simulink model "unpack"  (R2018b)
settings: Solver=VariableStepAuto  StartTime=0.0  StopTime=10.0  RelTol=1e-3
(part 2 of 2)

== matlab function unpack/message_unpack ==
  data: CAFDva_y_F_RadarData151 input size=22; CAFDva_y_F_RadarData152 input size=50; CAFDva_y_F_RadarData153 input size=50; CAFDva_y_F_RadarData154 input size=50; CAFDva_y_F_RadarData155 input size=50; CAFDva_y_F_RadarData156 input size=50; CAFDva_y_F_RadarData157 input size=50; CAFDva_y_F_RadarData158 input size=50; CAFDva_y_F_RadarData159 input size=50; CAFDva_y_F_RadarData15A input size=50; CAFDva_y_F_RadarData15B input size=50; CAFDva_y_F_RadarData15C input size=50; CAFDva_y_F_RadarData15D input size=50; CAFDva_y_F_RadarData15E input size=50; CAFDva_y_F_RadarData15F input size=50; CAFDva_y_F_RadarData160 input size=50; CAFDva_y_F_RadarData161 input size=50; CAFDva_y_F_RadarData162 input size=50; CAFDva_y_F_RadarData163 input size=50; CAFDva_y_F_RadarData164 input size=50; CAFDva_y_F_RadarData165 input size=50; CAFDva_y_F_RadarData166 input size=50; CAFDva_y_F_RadarData167 input size=50; CAFDva_y_F_RadarData168 input size=50; CAFDva_y_F_RadarData169 input size=50; CAFDva_y_F_CameraData600 input; CAFDva_y_F_CameraData424 input; CAFDva_y_F_CameraData425 input; CAFDva_y_F_CameraData450 input; CAFDva_y_F_CameraData459 input; CAFDva_y_F_CameraData45A input; CAFDva_y_F_CameraData45B input; CAFDva_y_F_CameraData45C input; CAFDva_y_F_CameraData45D input; CAFDva_y_F_CameraData45E input; CAFDva_y_F_CameraData45F input; CAFDva_y_F_CameraData420 input; CAFDva_y_F_CameraData421 input; CAFDva_y_F_CameraData422 input; CAFDva_y_F_CameraData451 input; CAFDva_y_F_CameraData423 input; CAFDva_y_F_CameraData452 input; CAFDva_y_F_CameraData453 input; CAFDva_y_F_CameraData454 input; CAFDva_y_F_CameraData455 input; CAFDva_y_F_CameraData456 input; CAFDva_y_F_CameraData457 input; CAFDva_y_F_CameraData458 input; CAFDva_y_F_CameraData449 input; Rar_obj_timestamp output; Radar_Status output; Radar_num output; CorrCoeff_x_vx output; CorrCoeff_y_vy output; CorrCoeff_y_vx output; CorrCoeff_x_vy output; IsNew output; YawSTD output; YawAngle output; WidthSTD output; Width output; RadarCrossSection output single; MovementStatus output; LongDistanceSTD output; LengthSTD output; Length output; LateralDistanceSTD output; LatDistance output; ExistenceProb output; CorrCoeff_x_y output; ClassType output; ClassProbValue output; CorrCoeff_vx_vy output; AbsoluteLongVelo output; AbsoluteLongAcc output; AbsoluteLatVelo output; AbsoluteLatAcc output; AbsLongVeloSTD output; AbsLongAccSTD output; AbsLatVeloSTD output; AbsLatAccSTD output; LongDistance output; ReferencePoint output; MeasurementStatus output; ObjectAge output; ObjectID output; IFC_obj_timestamp output; IFC_State output; IFC_ObjHdr_ObjCount output; IFC_VD_CIPV_ID output; FS_Out_Of_Calib output uint8; FS_Rain output; FS_Fog output; FS_Splashes_0 output; FS_Sun_Ray_0 output; FS_Low_Sun_0 output; FS_Blur_Image_0 output; FS_Partial_Blockage_0 output; FS_Full_Blockage_0 output; FS_Frozen_Windshield_0 output; FS_Out_Of_Focus_0 output; IFC_obj_TTIPC_StdDev output single; IFC_obj_abs_Ax output single; IFC_obj_abs_Ay output single; IFC_obj_Rel_Vx output; IFC_obj_Rel_Vy output; IFC_obj_Dx output; IFC_obj_Dy output single; IFC_obj_abs_AxStdDev output single; IFC_obj_abs_AyStdDev output single; IFC_obj_Rel_VxStdDev output single; IFC_obj_Rel_VyStdDev output single; IFC_obj_DxStdDev output single; IFC_obj_DyStdDev output single; IFC_obj_Rel_VxValid output uint8; IFC_obj_Rel_VyValid output uint8; IFC_obj_Rel_VxStdDevValid output uint8; IFC_obj_Rel_VyStdDevValid output uint8; IFC_obj_ExistProb output; IFC_obj_TypeProb output; IFC_obj_Width output; IFC_obj_Height output single; IFC_obj_LengthStdDev output single; IFC_obj_WidthStdDev output single; IFC_obj_HeightStdDev output single; IFC_obj_PhiLeft output; IFC_obj_PhiRight output; IFC_obj_angle_3D output single; IFC_obj_PhiLeftStdDev output single; IFC_obj_PhiRightStdDev output single; IFC_obj_angle_3DStdDev output single; IFC_obj_angle_rate output single; IFC_obj_angle_rate_StdDev output single; IFC_obj_PhiBottom output single; IFC_obj_PhiBottomStdDev output single; IFC_obj_Measured output uint8; IFC_obj_Heading output single; IFC_obj_HeadingStdDev output single; IFC_obj_HeadOrientation output uint8; IFC_obj_Type output; IFC_obj_ID output; IFC_obj_TTIPC output single; IFC_obj_DirIndicator output uint8; IFC_obj_BrakeLight output; IFC_Line01_LineID output; IFC_Line01_ExistProb output; IFC_Line01_DxStart output; IFC_Line01_ColorClass output; IFC_Line01_DxEnd output; IFC_Line01_HeadingAngle output; IFC_Line01_Dy output; IFC_Line01_CurvChange output; IFC_Line01_Curv output; IFC_Line01_MeasureType output; IFC_Line01_LineWidth output; IFC_Line01_Type output; IFC_Line01_TypeConf output; IFC_Line02_LineID output; IFC_Line02_ExistProb output; IFC_Line02_DxStart output; IFC_Line02_ColorClass output; IFC_Line02_DxEnd output; IFC_Line02_HeadingAngle output; IFC_Line02_Dy output; IFC_Line02_CurvChange output; IFC_Line02_Curv output; IFC_Line02_MeasureType output; IFC_Line02_LineWidth output; IFC_Line02_Type output; IFC_Line02_TypeConf output; IFC_Line03_LineID output; IFC_Line03_ExistProb output; IFC_Line03_DxStart output; IFC_Line03_ColorClass output; IFC_Line03_DxEnd output; IFC_Line03_HeadingAngle output; IFC_Line03_Dy output; IFC_Line03_CurvChange output; IFC_Line03_Curv output; IFC_Line03_MeasureType output; IFC_Line03_LineWidth output; IFC_Line03_Type output; IFC_Line03_TypeConf output; IFC_Line04_LineID output; IFC_Line04_ExistProb output; IFC_Line04_DxStart output; IFC_Line04_ColorClass output; IFC_Line04_DxEnd output; IFC_Line04_HeadingAngle output; IFC_Line04_Dy output; IFC_Line04_CurvChange output; IFC_Line04_Curv output; IFC_Line04_MeasureType output; IFC_Line04_LineWidth output; IFC_Line04_Type output; IFC_Line04_TypeConf output; IFC_Roadedge01_LineID output; IFC_Roadedge01_ExistProb output; IFC_Roadedge01_DxStart output; IFC_Roadedge01_DxEnd output; IFC_Roadedge01_HeadingAngle output; IFC_Roadedge01_Dy output; IFC_Roadedge01_Curv output; IFC_Roadedge01_CurvChange output; IFC_Roadedge01_MeasureType output; IFC_Roadedge01_Type output; IFC_Roadedge02_LineID output; IFC_Roadedge02_ExistProb output; IFC_Roadedge02_DxStart output; IFC_Roadedge02_DxEnd output; IFC_Roadedge02_HeadingAngle output; IFC_Roadedge02_Dy output; IFC_Roadedge02_Curv output; IFC_Roadedge02_CurvChange output; IFC_Roadedge02_MeasureType output; IFC_Roadedge02_Type output; IFC_obj_Length output; IFC_obj_Motion_Status output; IFC_obj_Lane_Assignment output; IFC_obj_Age output; IFC_obj_Rel_AxStdDev output; IFC_obj_Rel_Ax output; LH_Snown_Road_Prob output; COM_Is_ghSpeed_Road_V output; COM_Is_ghSpeed_Road output; LAP_Is_ghway_Merge_Right output; LAP_Is_ghway_Merge_Left output; LAP_Is_ghway_Exit_Right output; LAP_Is_ghway_Exit_Left output; LAP_Is_nstruction_Area output; OBJ_VRUount output; OBJ_VD_unt output; OBJ_Anil_Count output; ISA_Value output; ISA_Sign_Type output; ISA_Status output; ISA_Popup_text output; TSR_Vision_Only_Sign_Type output; ADAS_IHBC_High_Beam_Req output; ADAS_IHBC_Fuction_Status output; Radar_FaultBitSetting output; IFC_Lane1_C1 output; IFC_Lane2_C1 output; IFC_Lane3_C1 output; IFC_Lane4_C1 output; CAFDva_y_F_CameraData47E input; CAFDva_y_F_CameraData419 input; CAFDva_y_F_CameraData329 input; CAFDva_y_F_RadarData150 input; AEB_VD_Alert output; AEB_VD_ID output; AEB_VRU_Alert output; AEB_VRU_PED_ID output; AEBJA_VD_Alert output; AEBJA_VD_ID output; AEBJA_VRU_Alert output; AEBJA_VRU_PED_ID output; AEBPrefill_VRU_Alert output; AEBPrefill_VRU_PED_ID output; FCW_VD_Alert output; FCW_VD_ID output; FCW_VRU_Alert output; FCW_VRU_PED_ID output; JAPreFill_VD_Alert output; JAPreFill_VD_ID output; JAPreFill_VRU_Alert output; JAPreFill_VRU_PED_ID output
%% function for unpack and repack of canfd log data by liuyij 20210224
function [Rar_obj_timestamp,Radar_Status,Radar_num,...
    CorrCoeff_x_vx,CorrCoeff_y_vy,CorrCoeff_y_vx,CorrCoeff_x_vy,IsNew,YawSTD,YawAngle,...
    WidthSTD,Width,RadarCrossSection,MovementStatus,LongDistanceSTD,LengthSTD,Length,LateralDistanceSTD,LatDistance,...
    ExistenceProb,CorrCoeff_x_y,ClassType,ClassProbValue,CorrCoeff_vx_vy,AbsoluteLongVelo,AbsoluteLongAcc,AbsoluteLatVelo,...
    AbsoluteLatAcc,AbsLongVeloSTD,AbsLongAccSTD,AbsLatVeloSTD,AbsLatAccSTD,LongDistance,ReferencePoint,MeasurementStatus,ObjectAge,ObjectID,...
    IFC_obj_timestamp,IFC_State,IFC_ObjHdr_ObjCount,IFC_VD_CIPV_ID,...
    FS_Out_Of_Calib,FS_Rain,FS_Fog,FS_Splashes_0,FS_Sun_Ray_0,FS_Low_Sun_0,FS_Blur_Image_0,FS_Partial_Blockage_0,FS_Full_Blockage_0,FS_Frozen_Windshield_0,FS_Out_Of_Focus_0,...
    IFC_obj_TTIPC_StdDev,IFC_obj_abs_Ax,IFC_obj_abs_Ay,IFC_obj_Rel_Vx,IFC_obj_Rel_Vy,IFC_obj_Dx,IFC_obj_Dy,IFC_obj_abs_AxStdDev,IFC_obj_abs_AyStdDev,...
    IFC_obj_Rel_VxStdDev,IFC_obj_Rel_VyStdDev,IFC_obj_DxStdDev,IFC_obj_DyStdDev,IFC_obj_Rel_VxValid,IFC_obj_Rel_VyValid,IFC_obj_Rel_VxStdDevValid,...
    IFC_obj_Rel_VyStdDevValid,IFC_obj_ExistProb,IFC_obj_TypeProb,IFC_obj_Width,IFC_obj_Height,IFC_obj_LengthStdDev,IFC_obj_WidthStdDev,IFC_obj_HeightStdDev,...
    IFC_obj_PhiLeft,IFC_obj_PhiRight,IFC_obj_angle_3D,IFC_obj_PhiLeftStdDev,IFC_obj_PhiRightStdDev,IFC_obj_angle_3DStdDev,IFC_obj_angle_rate,...
    IFC_obj_angle_rate_StdDev,IFC_obj_PhiBottom,IFC_obj_PhiBottomStdDev,IFC_obj_Measured,IFC_obj_Heading,IFC_obj_HeadingStdDev,IFC_obj_HeadOrientation,...
    IFC_obj_Type,IFC_obj_ID,IFC_obj_TTIPC,IFC_obj_DirIndicator,IFC_obj_BrakeLight,...
    IFC_Line01_LineID,IFC_Line01_ExistProb,IFC_Line01_DxStart,IFC_Line01_ColorClass,IFC_Line01_DxEnd,IFC_Line01_HeadingAngle,IFC_Line01_Dy,...
    IFC_Line01_CurvChange,IFC_Line01_Curv,IFC_Line01_MeasureType,IFC_Line01_LineWidth,IFC_Line01_Type,IFC_Line01_TypeConf,...
    IFC_Line02_LineID,IFC_Line02_ExistProb,IFC_Line02_DxStart,IFC_Line02_ColorClass,IFC_Line02_DxEnd,IFC_Line02_HeadingAngle,IFC_Line02_Dy,...
    IFC_Line02_CurvChange,IFC_Line02_Curv,IFC_Line02_MeasureType,IFC_Line02_LineWidth,IFC_Line02_Type,IFC_Line02_TypeConf,...
    IFC_Line03_LineID,IFC_Line03_ExistProb,IFC_Line03_DxStart,IFC_Line03_ColorClass,IFC_Line03_DxEnd,IFC_Line03_HeadingAngle,IFC_Line03_Dy,...
    IFC_Line03_CurvChange,IFC_Line03_Curv,IFC_Line03_MeasureType,IFC_Line03_LineWidth,IFC_Line03_Type,IFC_Line03_TypeConf,...
    IFC_Line04_LineID,IFC_Line04_ExistProb,IFC_Line04_DxStart,IFC_Line04_ColorClass,IFC_Line04_DxEnd,IFC_Line04_HeadingAngle,IFC_Line04_Dy,...
    IFC_Line04_CurvChange,IFC_Line04_Curv,IFC_Line04_MeasureType,IFC_Line04_LineWidth,IFC_Line04_Type,IFC_Line04_TypeConf,...
    IFC_Roadedge01_LineID,IFC_Roadedge01_ExistProb,IFC_Roadedge01_DxStart,IFC_Roadedge01_DxEnd,IFC_Roadedge01_HeadingAngle,...
    IFC_Roadedge01_Dy,IFC_Roadedge01_Curv,IFC_Roadedge01_CurvChange,IFC_Roadedge01_MeasureType,IFC_Roadedge01_Type,...
    IFC_Roadedge02_LineID,IFC_Roadedge02_ExistProb,IFC_Roadedge02_DxStart,IFC_Roadedge02_DxEnd,IFC_Roadedge02_HeadingAngle,...
    IFC_Roadedge02_Dy,IFC_Roadedge02_Curv,IFC_Roadedge02_CurvChange,IFC_Roadedge02_MeasureType,IFC_Roadedge02_Type,...
    IFC_obj_Length,IFC_obj_Motion_Status,IFC_obj_Lane_Assignment,IFC_obj_Age,IFC_obj_Rel_AxStdDev,IFC_obj_Rel_Ax,...
    LH_Snown_Road_Prob,COM_Is_ghSpeed_Road_V,COM_Is_ghSpeed_Road,LAP_Is_ghway_Merge_Right,LAP_Is_ghway_Merge_Left,...
    LAP_Is_ghway_Exit_Right,LAP_Is_ghway_Exit_Left,LAP_Is_nstruction_Area,OBJ_VRUount,OBJ_VD_unt,OBJ_Anil_Count,...
    ISA_Value,ISA_Sign_Type,ISA_Status,ISA_Popup_text,TSR_Vision_Only_Sign_Type,ADAS_IHBC_High_Beam_Req,...
    ADAS_IHBC_Fuction_Status,Radar_FaultBitSetting,IFC_Lane1_C1,IFC_Lane2_C1,IFC_Lane3_C1,IFC_Lane4_C1,...
    AEB_VD_Alert,AEB_VD_ID,AEB_VRU_Alert,AEB_VRU_PED_ID,AEBJA_VD_Alert,AEBJA_VD_ID,AEBJA_VRU_Alert,AEBJA_VRU_PED_ID,...
    AEBPrefill_VRU_Alert,AEBPrefill_VRU_PED_ID,FCW_VD_Alert,FCW_VD_ID,FCW_VRU_Alert,FCW_VRU_PED_ID,...
    JAPreFill_VD_Alert,JAPreFill_VD_ID,JAPreFill_VRU_Alert,JAPreFill_VRU_PED_ID] ...
    = sensor_unpack(CAFDva_y_F_RadarData151,CAFDva_y_F_RadarData152,CAFDva_y_F_RadarData153,CAFDva_y_F_RadarData154,...
    CAFDva_y_F_RadarData155,CAFDva_y_F_RadarData156,CAFDva_y_F_RadarData157,CAFDva_y_F_RadarData158,CAFDva_y_F_RadarData159,...
    CAFDva_y_F_RadarData15A,CAFDva_y_F_RadarData15B,CAFDva_y_F_RadarData15C,CAFDva_y_F_RadarData15D,CAFDva_y_F_RadarData15E,CAFDva_y_F_RadarData15F,...
    CAFDva_y_F_RadarData160,CAFDva_y_F_RadarData161,CAFDva_y_F_RadarData162,CAFDva_y_F_RadarData163,CAFDva_y_F_RadarData164,...
    CAFDva_y_F_RadarData165,CAFDva_y_F_RadarData166,CAFDva_y_F_RadarData167,CAFDva_y_F_RadarData168,CAFDva_y_F_RadarData169,...
    CAFDva_y_F_CameraData600,CAFDva_y_F_CameraData424,CAFDva_y_F_CameraData425,CAFDva_y_F_CameraData450,CAFDva_y_F_CameraData459,...
    CAFDva_y_F_CameraData45A,CAFDva_y_F_CameraData45B,CAFDva_y_F_CameraData45C,CAFDva_y_F_CameraData45D,CAFDva_y_F_CameraData45E,...
    CAFDva_y_F_CameraData45F,CAFDva_y_F_CameraData420,CAFDva_y_F_CameraData421,CAFDva_y_F_CameraData422,CAFDva_y_F_CameraData451,...
    CAFDva_y_F_CameraData423,CAFDva_y_F_CameraData452,CAFDva_y_F_CameraData453,CAFDva_y_F_CameraData454,CAFDva_y_F_CameraData455,...
    CAFDva_y_F_CameraData456,CAFDva_y_F_CameraData457,CAFDva_y_F_CameraData458,CAFDva_y_F_CameraData449,CAFDva_y_F_CameraData47E,...
    CAFDva_y_F_CameraData419,CAFDva_y_F_CameraData329,CAFDva_y_F_RadarData150)

RADAR_MAX = uint8(24);
CAM_MAX = uint8(20);

%% output data initial 
% radar output
Radar_num = zeros(1,1,'uint8');
ObjectListQuali_ODH = zeros(1,1,'uint8');
Radar_Status = zeros(1,1,'uint8');
Radar_FaultBitSetting  = zeros(1,1,'uint8');

CorrCoeff_x_vx = zeros(RADAR_MAX,1,'single');
CorrCoeff_y_vy = zeros(RADAR_MAX,1,'single');
CorrCoeff_y_vx = zeros(RADAR_MAX,1,'single');
CorrCoeff_x_vy = zeros(RADAR_MAX,1,'single');
IsNew = zeros(RADAR_MAX,1,'uint8');
YawSTD = zeros(RADAR_MAX,1,'single');
YawAngle = zeros(RADAR_MAX,1,'single');
WidthSTD = zeros(RADAR_MAX,1,'single');
Width = zeros(RADAR_MAX,1,'single');
RadarCrossSection = zeros(RADAR_MAX,1,'single');
MovementStatus = zeros(RADAR_MAX,1,'uint8');
LongDistanceSTD = zeros(RADAR_MAX,1,'single');
LengthSTD = zeros(RADAR_MAX,1,'single');
Length = zeros(RADAR_MAX,1,'single');
LateralDistanceSTD = zeros(RADAR_MAX,1,'single');
LatDistance = zeros(RADAR_MAX,1,'single');
ExistenceProb = zeros(RADAR_MAX,1,'uint8');
CorrCoeff_x_y = zeros(RADAR_MAX,1,'single');
ClassType = zeros(RADAR_MAX,1,'uint8');
ClassProbValue = zeros(RADAR_MAX,1,'uint8');
CorrCoeff_vx_vy = zeros(RADAR_MAX,1,'single');
AbsoluteLongVelo = zeros(RADAR_MAX,1,'single');
AbsoluteLongAcc = zeros(RADAR_MAX,1,'single');
AbsoluteLatVelo = zeros(RADAR_MAX,1,'single');
AbsoluteLatAcc = zeros(RADAR_MAX,1,'single');
AbsLongVeloSTD = zeros(RADAR_MAX,1,'single');
AbsLongAccSTD = zeros(RADAR_MAX,1,'single');
AbsLatVeloSTD = zeros(RADAR_MAX,1,'single');
AbsLatAccSTD = zeros(RADAR_MAX,1,'single');
LongDistance = zeros(RADAR_MAX,1,'single');
ReferencePoint = zeros(RADAR_MAX,1,'uint8');
MeasurementStatus = zeros(RADAR_MAX,1,'uint8');
ObjectAge = zeros(RADAR_MAX,1,'single');
ObjectID = zeros(RADAR_MAX,1,'uint8');

Rar_obj_timestamp = zeros(RADAR_MAX,1,'uint16');

% cam output
IFC_State = zeros(1,1,'uint8');
IFC_ObjHdr_ObjCount = zeros(1,1,'uint8');
IFC_VD_CIPV_ID = zeros(1,1,'uint8');

FS_Out_Of_Calib = zeros(1,1,'uint8');
FS_Rain = zeros(1,1,'uint8');
FS_Fog = zeros(1,1,'uint8');
FS_Splashes_0 = zeros(1,1,'uint8');
FS_Sun_Ray_0 = zeros(1,1,'uint8');
FS_Low_Sun_0 = zeros(1,1,'uint8');
FS_Blur_Image_0 = zeros(1,1,'uint8');
FS_Partial_Blockage_0 = zeros(1,1,'uint8');
FS_Full_Blockage_0 = zeros(1,1,'uint8');
FS_Frozen_Windshield_0 = zeros(1,1,'uint8');
FS_Out_Of_Focus_0 = zeros(1,1,'uint8');

ISA_Value = zeros(1,1,'uint8');
ISA_Sign_Type = zeros(1,1,'uint8');
ISA_Status = zeros(1,1,'uint8');
ISA_Popup_text = zeros(1,1,'uint8');
TSR_Vision_Only_Sign_Type = zeros(1,1,'uint8');
ADAS_IHBC_High_Beam_Req = zeros(1,1,'uint8');
ADAS_IHBC_Fuction_Status = zeros(1,1,'uint8');


%% SW4.8 DF added--------------------------------
IFC_obj_Motion_Status = zeros(CAM_MAX,1,'uint8');
IFC_obj_Lane_Assignment = zeros(CAM_MAX,1,'uint8');
IFC_obj_Age = zeros(CAM_MAX,1,'uint16');
IFC_obj_Rel_AxStdDev = zeros(CAM_MAX,1,'single');
IFC_obj_Rel_Ax = zeros(CAM_MAX,1,'single');

LH_Snown_Road_Prob = zeros(1,1,'single');
COM_Is_ghSpeed_Road_V = zeros(1,1,'uint8');
COM_Is_ghSpeed_Road = zeros(1,1,'uint8');
LAP_Is_ghway_Merge_Right = zeros(1,1,'uint8');
LAP_Is_ghway_Merge_Left = zeros(1,1,'uint8');
LAP_Is_ghway_Exit_Right = zeros(1,1,'uint8');
LAP_Is_ghway_Exit_Left = zeros(1,1,'uint8');
LAP_Is_nstruction_Area = zeros(1,1,'uint8');

OBJ_VRUount = zeros(1,1,'uint8');
OBJ_VD_unt = zeros(1,1,'uint8');
OBJ_VD_PV_ID = zeros(1,1,'uint8');
OBJ_Anil_Count = zeros(1,1,'uint8');
%%-------------------------------------------------

IFC_obj_TTIPC_StdDev = zeros(CAM_MAX,1,'single');
IFC_obj_abs_Ax = zeros(CAM_MAX,1,'single');
IFC_obj_abs_Ay = zeros(CAM_MAX,1,'single');
IFC_obj_Rel_Vx = zeros(CAM_MAX,1,'single');
IFC_obj_Rel_Vy = zeros(CAM_MAX,1,'single');
IFC_obj_Dx = zeros(CAM_MAX,1,'single');
IFC_obj_Dy = zeros(CAM_MAX,1,'single');
IFC_obj_abs_AxStdDev = zeros(CAM_MAX,1,'single');
IFC_obj_abs_AyStdDev = zeros(CAM_MAX,1,'single');
IFC_obj_Rel_VxStdDev = zeros(CAM_MAX,1,'single');
IFC_obj_Rel_VyStdDev = zeros(CAM_MAX,1,'single');
IFC_obj_DxStdDev = zeros(CAM_MAX,1,'single');
IFC_obj_DyStdDev = zeros(CAM_MAX,1,'single');
IFC_obj_Rel_VxValid = zeros(CAM_MAX,1,'uint8');
IFC_obj_Rel_VyValid = zeros(CAM_MAX,1,'uint8');
IFC_obj_Rel_VxStdDevValid = zeros(CAM_MAX,1,'uint8');
IFC_obj_Rel_VyStdDevValid = zeros(CAM_MAX,1,'uint8');
IFC_obj_ExistProb = zeros(CAM_MAX,1,'single');
IFC_obj_TypeProb = zeros(CAM_MAX,1,'single');
IFC_obj_Length = zeros(CAM_MAX,1,'single');
IFC_obj_Width = zeros(CAM_MAX,1,'single');
IFC_obj_Height = zeros(CAM_MAX,1,'single');
IFC_obj_LengthStdDev = zeros(CAM_MAX,1,'single');
IFC_obj_WidthStdDev = zeros(CAM_MAX,1,'single');
IFC_obj_HeightStdDev = zeros(CAM_MAX,1,'single');
IFC_obj_PhiLeft = zeros(CAM_MAX,1,'single');
IFC_obj_PhiRight = zeros(CAM_MAX,1,'single');
IFC_obj_angle_3D = zeros(CAM_MAX,1,'single');
IFC_obj_PhiLeftStdDev = zeros(CAM_MAX,1,'single');
IFC_obj_PhiRightStdDev = zeros(CAM_MAX,1,'single');
IFC_obj_angle_3DStdDev = zeros(CAM_MAX,1,'single');
IFC_obj_angle_rate = zeros(CAM_MAX,1,'single');
IFC_obj_angle_rate_StdDev = zeros(CAM_MAX,1,'single');
IFC_obj_PhiBottom = zeros(CAM_MAX,1,'single');
IFC_obj_PhiBottomStdDev = zeros(CAM_MAX,1,'single');
IFC_obj_Measured = zeros(CAM_MAX,1,'uint8');
IFC_obj_Heading = zeros(CAM_MAX,1,'single');
IFC_obj_HeadingStdDev = zeros(CAM_MAX,1,'single');
IFC_obj_HeadOrientation = zeros(CAM_MAX,1,'uint8');
IFC_obj_Type = zeros(CAM_MAX,1,'uint8');
IFC_obj_ID = zeros(CAM_MAX,1,'uint8');
IFC_obj_TTIPC = zeros(CAM_MAX,1,'single');
IFC_obj_DirIndicator = zeros(CAM_MAX,1,'uint8');
IFC_obj_BrakeLight = zeros(CAM_MAX,1,'uint8');

IFC_obj_timestamp = zeros(CAM_MAX,1,'uint16');

IFC_Line01_LineID = zeros(1,1,'uint8');
IFC_Line01_ExistProb = zeros(1,1,'single');
IFC_Line01_DxStart = zeros(1,1,'single');
IFC_Line01_ColorClass = zeros(1,1,'uint8');
IFC_Line01_DxEnd = zeros(1,1,'single');
IFC_Line01_HeadingAngle = zeros(1,1,'single');
IFC_Line01_Dy = zeros(1,1,'single');
IFC_Line01_CurvChange = zeros(1,1,'single');
IFC_Line01_Curv = zeros(1,1,'single');
IFC_Line01_MeasureType = zeros(1,1,'uint8');
IFC_Line01_LineWidth = zeros(1,1,'single');
IFC_Line01_Type = zeros(1,1,'uint8');
IFC_Line01_TypeConf = zeros(1,1,'single');
IFC_Line02_LineID = zeros(1,1,'uint8');
IFC_Line02_ExistProb = zeros(1,1,'single');
IFC_Line02_DxStart = zeros(1,1,'single');
IFC_Line02_ColorClass = zeros(1,1,'uint8');
IFC_Line02_DxEnd = zeros(1,1,'single');
IFC_Line02_HeadingAngle = zeros(1,1,'single');
IFC_Line02_Dy = zeros(1,1,'single');
IFC_Line02_CurvChange = zeros(1,1,'single');
IFC_Line02_Curv = zeros(1,1,'single');
IFC_Line02_MeasureType = zeros(1,1,'uint8');
IFC_Line02_LineWidth = zeros(1,1,'single');
IFC_Line02_Type = zeros(1,1,'uint8');
IFC_Line02_TypeConf = zeros(1,1,'single');
IFC_Lane1_C1 = zeros(1,1,'single'); 
IFC_Lane2_C1 = zeros(1,1,'single'); 

IFC_Line03_LineID = zeros(1,1,'uint8');
IFC_Line03_ExistProb = zeros(1,1,'single');
IFC_Line03_DxStart = zeros(1,1,'single');
IFC_Line03_ColorClass = zeros(1,1,'uint8');
IFC_Line03_DxEnd = zeros(1,1,'single');
IFC_Line03_HeadingAngle = zeros(1,1,'single');
IFC_Line03_Dy = zeros(1,1,'single');
IFC_Line03_CurvChange = zeros(1,1,'single');
IFC_Line03_Curv = zeros(1,1,'single');
IFC_Line03_MeasureType = zeros(1,1,'uint8');
IFC_Line03_LineWidth = zeros(1,1,'single');
IFC_Line03_Type = zeros(1,1,'uint8');
IFC_Line03_TypeConf = zeros(1,1,'single');
IFC_Line04_LineID = zeros(1,1,'uint8');
IFC_Line04_ExistProb = zeros(1,1,'single');
IFC_Line04_DxStart = zeros(1,1,'single');
IFC_Line04_ColorClass = zeros(1,1,'uint8');
IFC_Line04_DxEnd = zeros(1,1,'single');
IFC_Line04_HeadingAngle = zeros(1,1,'single');
IFC_Line04_Dy = zeros(1,1,'single');
IFC_Line04_CurvChange = zeros(1,1,'single');
IFC_Line04_Curv = zeros(1,1,'single');
IFC_Line04_MeasureType = zeros(1,1,'uint8');
IFC_Line04_LineWidth = zeros(1,1,'single');
IFC_Line04_Type = zeros(1,1,'uint8');
IFC_Line04_TypeConf = zeros(1,1,'single');
IFC_Lane3_C1 = zeros(1,1,'single'); 
IFC_Lane4_C1 = zeros(1,1,'single'); 


IFC_Roadedge01_LineID = zeros(1,1,'uint8');
IFC_Roadedge01_ExistProb = zeros(1,1,'single');
IFC_Roadedge01_DxStart = zeros(1,1,'single');
IFC_Roadedge01_DxEnd = zeros(1,1,'single');
IFC_Roadedge01_HeadingAngle = zeros(1,1,'single');
IFC_Roadedge01_Dy = zeros(1,1,'single');
IFC_Roadedge01_Curv = zeros(1,1,'single');
IFC_Roadedge01_CurvChange = zeros(1,1,'single');
IFC_Roadedge01_MeasureType = zeros(1,1,'uint8');
IFC_Roadedge01_Type = zeros(1,1,'uint8');
IFC_Roadedge02_LineID = zeros(1,1,'uint8');
IFC_Roadedge02_ExistProb = zeros(1,1,'single');
IFC_Roadedge02_DxStart = zeros(1,1,'single');
IFC_Roadedge02_DxEnd = zeros(1,1,'single');
IFC_Roadedge02_HeadingAngle = zeros(1,1,'single');
IFC_Roadedge02_Dy = zeros(1,1,'single');
IFC_Roadedge02_Curv = zeros(1,1,'single');
IFC_Roadedge02_CurvChange = zeros(1,1,'single');
IFC_Roadedge02_MeasureType = zeros(1,1,'uint8');
IFC_Roadedge02_Type = zeros(1,1,'uint8');
%% put input message into temp matrix 
Radar_propty = zeros(50,RADAR_MAX,'uint8');
Cam_propty = zeros(66,CAM_MAX,'uint8');

%% get radar header property
[ ObjectListQuali_ODH,Radar_num] = get_radar_header(CAFDva_y_F_RadarData151);

[Radar_Status,Radar_FaultBitSetting]=get_radar_status(CAFDva_y_F_RadarData150);
%% put radar canfd message into temp matrix 
Radar_propty = [CAFDva_y_F_RadarData152,CAFDva_y_F_RadarData153,CAFDva_y_F_RadarData154,CAFDva_y_F_RadarData155,...
    CAFDva_y_F_RadarData156,CAFDva_y_F_RadarData157,CAFDva_y_F_RadarData158,CAFDva_y_F_RadarData159,CAFDva_y_F_RadarData15A,...
    CAFDva_y_F_RadarData15B,CAFDva_y_F_RadarData15C,CAFDva_y_F_RadarData15D,CAFDva_y_F_RadarData15E,CAFDva_y_F_RadarData15F,...
    CAFDva_y_F_RadarData160,CAFDva_y_F_RadarData161,CAFDva_y_F_RadarData162,CAFDva_y_F_RadarData163,CAFDva_y_F_RadarData164,...
    CAFDva_y_F_RadarData165,CAFDva_y_F_RadarData166,CAFDva_y_F_RadarData167,CAFDva_y_F_RadarData168,CAFDva_y_F_RadarData169];
%% get radar obj property
[Rar_obj_timestamp,CorrCoeff_x_vx,CorrCoeff_y_vy,CorrCoeff_y_vx,CorrCoeff_x_vy,...
    IsNew,YawSTD,YawAngle,WidthSTD,Width,RadarCrossSection,MovementStatus,LongDistanceSTD,LengthSTD,Length,...
    LateralDistanceSTD,LatDistance,ExistenceProb,CorrCoeff_x_y,ClassType,ClassProbValue,CorrCoeff_vx_vy,...
    AbsoluteLongVelo,AbsoluteLongAcc,AbsoluteLatVelo,AbsoluteLatAcc,AbsLongVeloSTD,AbsLongAccSTD,AbsLatVeloSTD,...
    AbsLatAccSTD,LongDistance,ReferencePoint,MeasurementStatus,ObjectAge,ObjectID] = unpack_radar_obj_proty(Radar_propty,RADAR_MAX);

%% put cam canfd message into temp matrix 
Cam_propty =[CAFDva_y_F_CameraData450,CAFDva_y_F_CameraData451,CAFDva_y_F_CameraData452,CAFDva_y_F_CameraData453,...
    CAFDva_y_F_CameraData454,CAFDva_y_F_CameraData455,CAFDva_y_F_CameraData456,CAFDva_y_F_CameraData457,...
   CAFDva_y_F_CameraData458,CAFDva_y_F_CameraData459,CAFDva_y_F_CameraData45A,CAFDva_y_F_CameraData45B,...
    CAFDva_y_F_CameraData45C,CAFDva_y_F_CameraData45D,CAFDva_y_F_CameraData45E,CAFDva_y_F_CameraData45F,...
    CAFDva_y_F_CameraData420,CAFDva_y_F_CameraData421,CAFDva_y_F_CameraData422,CAFDva_y_F_CameraData423]; 
% %% get cam road property    
% [IFC_State,IFC_ObjHdr_ObjCount,IFC_VD_CIPV_ID] = unpack_cam_status(CAFDva_y_F_CameraData426);
[LH_Snown_Road_Prob,COM_Is_ghSpeed_Road_V,COM_Is_ghSpeed_Road,LAP_Is_ghway_Merge_Right,LAP_Is_ghway_Merge_Left,...
    LAP_Is_ghway_Exit_Right,LAP_Is_ghway_Exit_Left,LAP_Is_nstruction_Area] = unpack_cam_road_property(CAFDva_y_F_CameraData419);
% %% get cam num cipv property 
%  [OBJ_VRUount,OBJ_VD_unt,IFC_VD_CIPV_ID,OBJ_Anil_Count] = unpack_cam_num_cipv(CAFDva_y_F_CameraData449);
[OBJ_VRUount,OBJ_VD_unt,OBJ_VD_PV_ID,OBJ_Anil_Count,AEB_VD_Alert,AEB_VD_ID,...
    AEB_VRU_Alert,AEB_VRU_PED_ID,AEBJA_VD_Alert,AEBJA_VD_ID,AEBJA_VRU_Alert,AEBJA_VRU_PED_ID,...
    AEBPrefill_VRU_Alert,AEBPrefill_VRU_PED_ID,FCW_VD_Alert,FCW_VD_ID,FCW_VRU_Alert,FCW_VRU_PED_ID,...
    JAPreFill_VD_Alert,JAPreFill_VD_ID,JAPreFill_VRU_Alert,JAPreFill_VRU_PED_ID] = unpack_cam_num_cipv(CAFDva_y_F_CameraData449);
% %% get cam status
 [IFC_State,ISA_Value,ISA_Sign_Type,ISA_Status,ISA_Popup_text,TSR_Vision_Only_Sign_Type,ADAS_IHBC_High_Beam_Req,...
     ADAS_IHBC_Fuction_Status] = unpack_cam_status(CAFDva_y_F_CameraData329);
% %% get cam failsafe property
[FS_Out_Of_Calib,FS_Rain,FS_Fog,FS_Splashes_0,FS_Sun_Ray_0,FS_Low_Sun_0,FS_Blur_Image_0,FS_Partial_Blockage_0,...
    FS_Full_Blockage_0,FS_Frozen_Windshield_0,FS_Out_Of_Focus_0] = unpack_cam_failsafe(CAFDva_y_F_CameraData600);
%% get cam obj property
[IFC_obj_timestamp,IFC_obj_TTIPC_StdDev,IFC_obj_abs_Ax,IFC_obj_abs_Ay,IFC_obj_Rel_Vx,IFC_obj_Rel_Vy,IFC_obj_Dx,IFC_obj_Dy,...
    IFC_obj_abs_AxStdDev,IFC_obj_abs_AyStdDev,IFC_obj_Rel_VxStdDev,IFC_obj_Rel_VyStdDev,IFC_obj_DxStdDev,IFC_obj_DyStdDev,...
    IFC_obj_Rel_VxValid,IFC_obj_Rel_VyValid,IFC_obj_Rel_VxStdDevValid,IFC_obj_Rel_VyStdDevValid,IFC_obj_ExistProb,IFC_obj_TypeProb,...
    IFC_obj_Width,IFC_obj_Height,IFC_obj_LengthStdDev,IFC_obj_WidthStdDev,IFC_obj_HeightStdDev,IFC_obj_PhiLeft,IFC_obj_PhiRight,...
    IFC_obj_angle_3D,IFC_obj_PhiLeftStdDev,IFC_obj_PhiRightStdDev,IFC_obj_angle_3DStdDev,IFC_obj_angle_rate,IFC_obj_angle_rate_StdDev,...
    IFC_obj_PhiBottom,IFC_obj_PhiBottomStdDev,IFC_obj_Measured,IFC_obj_Heading,IFC_obj_HeadingStdDev,IFC_obj_HeadOrientation,IFC_obj_Type,...
    IFC_obj_ID,IFC_obj_TTIPC,IFC_obj_DirIndicator,IFC_obj_BrakeLight,IFC_obj_Motion_Status,IFC_obj_Lane_Assignment,IFC_obj_Age,...
    IFC_obj_Rel_AxStdDev,IFC_obj_Rel_Ax,IFC_obj_Length] = unpack_cam_obj_proty(Cam_propty,CAM_MAX);
%% get cam lane L0R0
[IFC_Line01_LineID,IFC_Line01_ExistProb,IFC_Line01_DxStart,IFC_Line01_ColorClass,IFC_Line01_DxEnd,IFC_Line01_HeadingAngle,IFC_Line01_Dy,...
    IFC_Line01_CurvChange,IFC_Line01_Curv,IFC_Line01_MeasureType,IFC_Line01_LineWidth,IFC_Line01_Type,IFC_Line01_TypeConf,...
    IFC_Line02_LineID,IFC_Line02_ExistProb,IFC_Line02_DxStart,IFC_Line02_ColorClass,IFC_Line02_DxEnd,IFC_Line02_HeadingAngle,IFC_Line02_Dy,...
    IFC_Line02_CurvChange,IFC_Line02_Curv,IFC_Line02_MeasureType,IFC_Line02_LineWidth,IFC_Line02_Type,IFC_Line02_TypeConf,...
IFC_Lane1_C1,IFC_Lane2_C1] = unpack_cam_L0R0(CAFDva_y_F_CameraData424);
%% get cam lane L1R1
[IFC_Line03_LineID,IFC_Line03_ExistProb,IFC_Line03_DxStart,IFC_Line03_ColorClass,IFC_Line03_DxEnd,IFC_Line03_HeadingAngle,IFC_Line03_Dy,...
    IFC_Line03_CurvChange,IFC_Line03_Curv,IFC_Line03_MeasureType,IFC_Line03_LineWidth,IFC_Line03_Type,IFC_Line03_TypeConf,...
    IFC_Line04_LineID,IFC_Line04_ExistProb,IFC_Line04_DxStart,IFC_Line04_ColorClass,IFC_Line04_DxEnd,IFC_Line04_HeadingAngle,IFC_Line04_Dy,...
    IFC_Line04_CurvChange,IFC_Line04_Curv,IFC_Line04_MeasureType,IFC_Line04_LineWidth,IFC_Line04_Type,IFC_Line04_TypeConf,...
IFC_Lane3_C1,IFC_Lane4_C1] = unpack_cam_L1R1(CAFDva_y_F_CameraData425);
%% get cam Roadedge
[IFC_Roadedge01_LineID,IFC_Roadedge01_ExistProb,IFC_Roadedge01_DxStart,IFC_Roadedge01_DxEnd,IFC_Roadedge01_HeadingAngle,...
    IFC_Roadedge01_Dy,IFC_Roadedge01_Curv,IFC_Roadedge01_CurvChange,IFC_Roadedge01_MeasureType,IFC_Roadedge01_Type,...
    IFC_Roadedge02_LineID,IFC_Roadedge02_ExistProb,IFC_Roadedge02_DxStart,IFC_Roadedge02_DxEnd,IFC_Roadedge02_HeadingAngle,...
    IFC_Roadedge02_Dy,IFC_Roadedge02_Curv,IFC_Roadedge02_CurvChange,IFC_Roadedge02_MeasureType,IFC_Roadedge02_Type...
] = unpack_cam_roadedge(CAFDva_y_F_CameraData47E);
end

function[radar_status,radar_faultbitsetting]=get_radar_status(radar_status_in)
radar_status = uint8(radar_status_in(3));
radar_faultbitsetting = uint8(radar_status_in(4));
if radar_status == uint8(7)
    radar_status = uint8(6);
end

if radar_status == uint8(8)
    radar_status = uint8(7);
end
end

function[radar_status,radar_obj_num]=get_radar_header(radar_header)
radar_status = bitshift(uint8(radar_header(18)),-5);
radar_obj_num = uint8(radar_header(19));
end

function [Rar_obj_timestamp,CorrCoeff_x_vx,CorrCoeff_y_vy,CorrCoeff_y_vx,CorrCoeff_x_vy,...
    IsNew,YawSTD,YawAngle,WidthSTD,Width,RadarCrossSection,MovementStatus,LongDistanceSTD,LengthSTD,Length,...
    LateralDistanceSTD,LatDistance,ExistenceProb,CorrCoeff_x_y,ClassType,ClassProbValue,CorrCoeff_vx_vy,...
    AbsoluteLongVelo,AbsoluteLongAcc,AbsoluteLatVelo,AbsoluteLatAcc,AbsLongVeloSTD,AbsLongAccSTD,AbsLatVeloSTD,...
    AbsLatAccSTD,LongDistance,ReferencePoint,MeasurementStatus,ObjectAge,ObjectID] = unpack_radar_obj_proty(Rar_obj,RADAR_MAX)

CorrCoeff_x_vx = zeros(RADAR_MAX,1,'single');
CorrCoeff_y_vy = zeros(RADAR_MAX,1,'single');
CorrCoeff_y_vx = zeros(RADAR_MAX,1,'single');
CorrCoeff_x_vy = zeros(RADAR_MAX,1,'single');
IsNew = zeros(RADAR_MAX,1,'uint8');
YawSTD = zeros(RADAR_MAX,1,'single');
YawAngle = zeros(RADAR_MAX,1,'single');
WidthSTD = zeros(RADAR_MAX,1,'single');
Width = zeros(RADAR_MAX,1,'single');
RadarCrossSection = zeros(RADAR_MAX,1,'single');
MovementStatus = zeros(RADAR_MAX,1,'uint8');
LongDistanceSTD = zeros(RADAR_MAX,1,'single');
LengthSTD = zeros(RADAR_MAX,1,'single');
Length = zeros(RADAR_MAX,1,'single');
LateralDistanceSTD = zeros(RADAR_MAX,1,'single');
LatDistance = zeros(RADAR_MAX,1,'single');
ExistenceProb = zeros(RADAR_MAX,1,'uint8');
CorrCoeff_x_y = zeros(RADAR_MAX,1,'single');
ClassType = zeros(RADAR_MAX,1,'uint8');
ClassProbValue = zeros(RADAR_MAX,1,'uint8');
CorrCoeff_vx_vy = zeros(RADAR_MAX,1,'single');
AbsoluteLongVelo = zeros(RADAR_MAX,1,'single');
AbsoluteLongAcc = zeros(RADAR_MAX,1,'single');
AbsoluteLatVelo = zeros(RADAR_MAX,1,'single');
AbsoluteLatAcc = zeros(RADAR_MAX,1,'single');
AbsLongVeloSTD = zeros(RADAR_MAX,1,'single');
AbsLongAccSTD = zeros(RADAR_MAX,1,'single');
AbsLatVeloSTD = zeros(RADAR_MAX,1,'single');
AbsLatAccSTD = zeros(RADAR_MAX,1,'single');
LongDistance = zeros(RADAR_MAX,1,'single');
ReferencePoint = zeros(RADAR_MAX,1,'uint8');
MeasurementStatus = zeros(RADAR_MAX,1,'uint8');
ObjectAge = zeros(RADAR_MAX,1,'single');
ObjectID = zeros(RADAR_MAX,1,'uint8');

Rar_obj_timestamp = zeros(RADAR_MAX,1,'uint16');

for i=1:RADAR_MAX
	CorrCoeff_x_vx(i) = single(fromBit_intel(81,8,Rar_obj(3:41,i)))*single(0.01)+single(-1.0);
	CorrCoeff_y_vy(i) = single(fromBit_intel(264,8,Rar_obj(3:41,i)))*single(0.01)+single(-1.0);
	CorrCoeff_y_vx(i) = single(fromBit_intel(256,8,Rar_obj(3:41,i)))*single(0.01)+single(-1.0);
	CorrCoeff_x_vy(i) = single(fromBit_intel(210,8,Rar_obj(3:41,i)))*single(0.01)+single(-1.0);
	IsNew(i) = uint8(fromBit_intel(24,2,Rar_obj(3:41,i)));
	YawSTD(i) = single(fromBit_intel(288,9,Rar_obj(3:41,i)))*single(0.02)+single(0.0);
	YawAngle(i) = single(fromBit_intel(279,9,Rar_obj(3:41,i)))*single(0.02)+single(-3.142);
	WidthSTD(i) = single(fromBit_intel(175,6,Rar_obj(3:41,i)))*single(0.1)+single(0.0);
	Width(i) = single(fromBit_intel(169,6,Rar_obj(3:41,i)))*single(0.1)+single(0.0);
	RadarCrossSection(i) = single(fromBit_intel(272,7,Rar_obj(3:41,i)))+single(-60);
	MovementStatus(i) = uint8(fromBit_intel(45,3,Rar_obj(3:41,i)));
	LongDistanceSTD(i) = single(fromBit_intel(239,9,Rar_obj(3:41,i)))*single(0.05)+single(0.0);
	LengthSTD(i) = single(fromBit_intel(142,7,Rar_obj(3:41,i)))*single(0.1)+single(0.0);
	Length(i) = single(fromBit_intel(248,8,Rar_obj(3:41,i)))*single(0.1)+single(0.0);
	LateralDistanceSTD(i) = single(fromBit_intel(230,9,Rar_obj(3:41,i)))*single(0.05)+single(0.0);
	LatDistance(i) = single(fromBit_intel(218,12,Rar_obj(3:41,i)))*single(0.05)+single(-100.0);
	ExistenceProb(i) = uint8(fromBit_intel(89,7,Rar_obj(3:41,i)));
	CorrCoeff_x_y(i) = single(fromBit_intel(202,8,Rar_obj(3:41,i)))*single(0.01)+single(-1.0);
	ClassType(i) = uint8(fromBit_intel(26,3,Rar_obj(3:41,i)));
	ClassProbValue(i) = uint8(fromBit_intel(105,7,Rar_obj(3:41,i)));
	CorrCoeff_vx_vy(i) = single(fromBit_intel(181,8,Rar_obj(3:41,i)))*single(0.01)+single(-1.0);
	AbsoluteLongVelo(i) = single(fromBit_intel(60,12,Rar_obj(3:41,i)))*single(0.05)+single(-100.0);
	AbsoluteLongAcc(i) = single(fromBit_intel(159,10,Rar_obj(3:41,i)))*single(0.05)+single(-25.0);
	AbsoluteLatVelo(i) = single(fromBit_intel(130,12,Rar_obj(3:41,i)))*single(0.05)+single(-100.0);
	AbsoluteLatAcc(i) = single(fromBit_intel(149,10,Rar_obj(3:41,i)))*single(0.05)+single(-25.0);
	AbsLongVeloSTD(i) = single(fromBit_intel(121,9,Rar_obj(3:41,i)))*single(0.02)+single(0.0);
	AbsLongAccSTD(i) = single(fromBit_intel(112,9,Rar_obj(3:41,i)))*single(0.008)+single(0.0);
	AbsLatVeloSTD(i) = single(fromBit_intel(96,9,Rar_obj(3:41,i)))*single(0.02)+single(0.0);
	AbsLatAccSTD(i) = single(fromBit_intel(72,9,Rar_obj(3:41,i)))*single(0.008)+single(0.0);
	LongDistance(i) = single(fromBit_intel(32,13,Rar_obj(3:41,i)))*single(0.05)+single(-50.0);
	ReferencePoint(i) = uint8(fromBit_intel(56,4,Rar_obj(3:41,i)));
	MeasurementStatus(i) = uint8(fromBit_intel(29,3,Rar_obj(3:41,i)));
	ObjectAge(i) = single(fromBit_intel(189,13,Rar_obj(3:41,i)))*single(0.06)+single(0.0);
	ObjectID(i) = uint8(fromBit_intel(48,8,Rar_obj(3:41,i)));
	Rar_obj_timestamp(i) =  bitor(bitshift(uint16(Rar_obj(1,i)),8),uint16(Rar_obj(2,i)));
end
end



%% intel format CANFD message unpack(without above timestamps)
function num  = fromBit_intel(startbit,length,all)
startbyte=(floor(startbit/8)+1); %%get row of message lsb
endbit=rem(startbit,8);        %%get column of message lsb
byte1=bitshift(uint32(all(startbyte)),-endbit);%%rightshift lsb row
byte2=bitshift(uint32(all(startbyte+1)),8-endbit);%%leftshift msb row
byte3=bitshift(uint32(all(startbyte+2)),16-endbit);%%leftshift msb row
num=uint32(bitand(bitor(bitor(byte1,byte2),byte3),pow2(length)-uint32(1))); %%merge and pick valid bit of data
end

%% intel IEEE float format CANFD message unpack(without above timestamps)
function num  = fromBit_intel_IEE_float(startbit,length,all)
startbyte=(floor(startbit/8)+1); %%get row of message lsb
endbit=rem(startbit,8);        %%get column of message lsb
byte1=bitshift(uint32(all(startbyte)),-endbit);%%rightshift lsb row
byte2=bitshift(uint32(all(startbyte+1)),8-endbit);%%leftshift msb row
byte3=bitshift(uint32(all(startbyte+2)),16-endbit);%%leftshift msb row
byte4=bitshift(uint32(all(startbyte+3)),24-endbit);%%leftshift msb row
% byte1=bitshift(uint32(all(startbyte)),24);%%rightshift lsb row
% byte2=bitshift(uint32(all(startbyte+1)),16);%%leftshift msb row
% byte3=bitshift(uint32(all(startbyte+2)),8);%%leftshift msb row
% byte4=bitshift(uint32(all(startbyte+3)),0);%%leftshift msb row
temp_num= bitor(bitor(bitor(byte1,byte2),byte3),byte4);
num_flag = single(bitget(temp_num,32));
point_sid = single(bitshift(bitshift(bitshift(temp_num,1),-1),-23))-single(127);
num = single((-1)^num_flag*(single(1)+single(bitshift(bitshift(temp_num,9),-9))*2^(-23))*2^point_sid);
end

%% motorola format CANFD message unpack(without above timestamps)    
function num  = fromBit_motorola(startbit,length,all)
startbyte =(floor(startbit/(8))+1);
endbit=rem((startbit),(8));
%%initial of byte3 and byte4
byte3 = uint32(0);
byte4 = uint32(0);
byte1=bitshift(uint32(all(startbyte)),-endbit);%右移
byte2=bitshift(uint32(all(startbyte-1)),8-endbit);%左移
if startbyte>uint8(3)
    byte3=bitshift(uint32(all(startbyte-2)),16-endbit);%左移
    byte4=bitshift(uint32(all(startbyte-3)),24-endbit);%左移
end
num=uint32(bitand(bitor(bitor(bitor(byte1,byte2),byte3),byte4),pow2(length)-uint32(1)));
end

%% motorola format CANFD message unpack(without above timestamps)    
function num  = fromBit_motorola_onelane(startbit,length,all)
startbyte =(floor(startbit/(8))+1);
endbit=rem((startbit),(8));
byte1=bitshift(uint32(all(startbyte)),-endbit);%右移
num=uint32(bitand(byte1,pow2(length)-uint32(1)));
end

function [IFC_obj_timestamp,IFC_obj_TTIPC_StdDev,IFC_obj_abs_Ax,IFC_obj_abs_Ay,IFC_obj_Rel_Vx,IFC_obj_Rel_Vy,IFC_obj_Dx,IFC_obj_Dy,IFC_obj_abs_AxStdDev,IFC_obj_abs_AyStdDev,IFC_obj_Rel_VxStdDev,IFC_obj_Rel_VyStdDev,IFC_obj_DxStdDev,IFC_obj_DyStdDev,IFC_obj_Rel_VxValid,IFC_obj_Rel_VyValid,IFC_obj_Rel_VxStdDevValid,IFC_obj_Rel_VyStdDevValid,IFC_obj_ExistProb,IFC_obj_TypeProb,IFC_obj_Width,IFC_obj_Height,IFC_obj_LengthStdDev,IFC_obj_WidthStdDev,IFC_obj_HeightStdDev,IFC_obj_PhiLeft,IFC_obj_PhiRight,IFC_obj_angle_3D,IFC_obj_PhiLeftStdDev,IFC_obj_PhiRightStdDev,IFC_obj_angle_3DStdDev,IFC_obj_angle_rate,IFC_obj_angle_rate_StdDev,IFC_obj_PhiBottom,IFC_obj_PhiBottomStdDev,IFC_obj_Measured,IFC_obj_Heading,IFC_obj_HeadingStdDev,IFC_obj_HeadOrientation,IFC_obj_Type,IFC_obj_ID,IFC_obj_TTIPC,IFC_obj_DirIndicator,IFC_obj_BrakeLight,...
IFC_obj_Motion_Status,IFC_obj_Lane_Assignment,IFC_obj_Age,IFC_obj_Rel_AxStdDev,IFC_obj_Rel_Ax,IFC_obj_Length] = unpack_cam_obj_proty(Cam_obj,CAM_MAX)

IFC_obj_Motion_Status = zeros(CAM_MAX,1,'uint8');
IFC_obj_Lane_Assignment = zeros(CAM_MAX,1,'uint8');
IFC_obj_Age = zeros(CAM_MAX,1,'uint16');
IFC_obj_Rel_AxStdDev = zeros(CAM_MAX,1,'single');
IFC_obj_Rel_Ax = zeros(CAM_MAX,1,'single');

IFC_obj_TTIPC_StdDev = zeros(CAM_MAX,1,'single');
IFC_obj_abs_Ax = zeros(CAM_MAX,1,'single');
IFC_obj_abs_Ay = zeros(CAM_MAX,1,'single');
IFC_obj_Rel_Vx = zeros(CAM_MAX,1,'single');
IFC_obj_Rel_Vy = zeros(CAM_MAX,1,'single');
IFC_obj_Dx = zeros(CAM_MAX,1,'single');
IFC_obj_Dy = zeros(CAM_MAX,1,'single');
IFC_obj_abs_AxStdDev = zeros(CAM_MAX,1,'single');
IFC_obj_abs_AyStdDev = zeros(CAM_MAX,1,'single');
IFC_obj_Rel_VxStdDev = zeros(CAM_MAX,1,'single');
IFC_obj_Rel_VyStdDev = zeros(CAM_MAX,1,'single');
IFC_obj_DxStdDev = zeros(CAM_MAX,1,'single');
IFC_obj_DyStdDev = zeros(CAM_MAX,1,'single');
IFC_obj_Rel_VxValid = zeros(CAM_MAX,1,'uint8');
IFC_obj_Rel_VyValid = zeros(CAM_MAX,1,'uint8');
IFC_obj_Rel_VxStdDevValid = zeros(CAM_MAX,1,'uint8');
IFC_obj_Rel_VyStdDevValid = zeros(CAM_MAX,1,'uint8');
IFC_obj_ExistProb = zeros(CAM_MAX,1,'single');
IFC_obj_TypeProb = zeros(CAM_MAX,1,'single');
IFC_obj_Length = zeros(CAM_MAX,1,'single');
IFC_obj_Width = zeros(CAM_MAX,1,'single');
IFC_obj_Height = zeros(CAM_MAX,1,'single');
IFC_obj_LengthStdDev = zeros(CAM_MAX,1,'single');
IFC_obj_WidthStdDev = zeros(CAM_MAX,1,'single');
IFC_obj_HeightStdDev = zeros(CAM_MAX,1,'single');
IFC_obj_PhiLeft = zeros(CAM_MAX,1,'single');
IFC_obj_PhiRight = zeros(CAM_MAX,1,'single');
IFC_obj_angle_3D = zeros(CAM_MAX,1,'single');
IFC_obj_PhiLeftStdDev = zeros(CAM_MAX,1,'single');
IFC_obj_PhiRightStdDev = zeros(CAM_MAX,1,'single');
IFC_obj_angle_3DStdDev = zeros(CAM_MAX,1,'single');
IFC_obj_angle_rate = zeros(CAM_MAX,1,'single');
IFC_obj_angle_rate_StdDev = zeros(CAM_MAX,1,'single');
IFC_obj_PhiBottom = zeros(CAM_MAX,1,'single');
IFC_obj_PhiBottomStdDev = zeros(CAM_MAX,1,'single');
IFC_obj_Measured = zeros(CAM_MAX,1,'uint8');
IFC_obj_Heading = zeros(CAM_MAX,1,'single');
IFC_obj_HeadingStdDev = zeros(CAM_MAX,1,'single');
IFC_obj_HeadOrientation = zeros(CAM_MAX,1,'uint8');
IFC_obj_Type = zeros(CAM_MAX,1,'uint8');
IFC_obj_ID = zeros(CAM_MAX,1,'uint8');
IFC_obj_TTIPC = zeros(CAM_MAX,1,'single');
IFC_obj_DirIndicator = zeros(CAM_MAX,1,'uint8');
IFC_obj_BrakeLight = zeros(CAM_MAX,1,'uint8');

IFC_obj_timestamp = zeros(CAM_MAX,1,'uint16');
for i=1:CAM_MAX
	IFC_obj_Motion_Status(i) = uint8(fromBit_intel(419,4,Cam_obj(3:66,i)));
	IFC_obj_Lane_Assignment(i) = uint8(fromBit_intel(451,3,Cam_obj(3:66,i)));
	IFC_obj_Age(i) = uint16(fromBit_intel(440,11,Cam_obj(3:66,i)));
	IFC_obj_Rel_AxStdDev(i) = single(fromBit_intel(432,8,Cam_obj(3:66,i)))*single(0.05)+single(0.0);
	IFC_obj_Rel_Ax(i) = single(fromBit_intel(423,9,Cam_obj(3:66,i)))*single(0.05)+single(-10.3);
	
	IFC_obj_abs_Ax(i) = single(fromBit_intel(352,9,Cam_obj(3:66,i)))*single(0.05)+single(-10.3);
	IFC_obj_abs_Ay(i) = single(fromBit_intel(39,9,Cam_obj(3:66,i)))*single(0.05)+single(-10.3);
	IFC_obj_Rel_Vx(i) = single(fromBit_intel(76,13,Cam_obj(3:66,i)))*single(0.05)+single(-120.0);
	IFC_obj_Rel_Vy(i) = single(fromBit_intel(192,11,Cam_obj(3:66,i)))*single(0.05)+single(-50.0);
	IFC_obj_Dx(i) = single(fromBit_intel(50,14,Cam_obj(3:66,i)))*single(0.05)+single(-200.0);
	IFC_obj_Dy(i) = single(fromBit_intel(64,12,Cam_obj(3:66,i)))*single(0.05)+single(-100.0);
	IFC_obj_abs_AxStdDev(i) = single(fromBit_intel(24,8,Cam_obj(3:66,i)))*single(0.05)+single(0.0);
	IFC_obj_abs_AyStdDev(i) = single(fromBit_intel(216,8,Cam_obj(3:66,i)))*single(0.05)+single(0.0);
	IFC_obj_Rel_VxStdDev(i) = single(fromBit_intel(169,11,Cam_obj(3:66,i)))*single(0.05)+single(0.0);
	IFC_obj_Rel_VyStdDev(i) = single(fromBit_intel(96,10,Cam_obj(3:66,i)))*single(0.05)+single(0.0);
	IFC_obj_DxStdDev(i) = single(fromBit_intel(115,13,Cam_obj(3:66,i)))*single(0.05)+single(0.0);
	IFC_obj_DyStdDev(i) = single(fromBit_intel(128,11,Cam_obj(3:66,i)))*single(0.05)+single(0.0);
	IFC_obj_Rel_VxValid(i) = uint8(fromBit_intel(48,1,Cam_obj(3:66,i)));
	IFC_obj_Rel_VyValid(i) = uint8(fromBit_intel(49,1,Cam_obj(3:66,i)));
	IFC_obj_Rel_VxStdDevValid(i) = uint8(fromBit_intel(319,1,Cam_obj(3:66,i)));
	IFC_obj_Rel_VyStdDevValid(i) = uint8(fromBit_intel(351,1,Cam_obj(3:66,i)));
	IFC_obj_ExistProb(i) = single(fromBit_intel(89,7,Cam_obj(3:66,i)))*single(0.01)+single(0.0);
	IFC_obj_TypeProb(i) = single(fromBit_intel(32,7,Cam_obj(3:66,i)))*single(0.01)+single(0.0);
	IFC_obj_Length(i) = single(fromBit_intel(160,9,Cam_obj(3:66,i)))*single(0.05)+single(1.2);
	IFC_obj_Width(i) = single(fromBit_intel(106,9,Cam_obj(3:66,i)))*single(0.01)+single(0.4);
	IFC_obj_Height(i) = single(fromBit_intel(288,9,Cam_obj(3:66,i)))*single(0.01)+single(0.0);
	IFC_obj_LengthStdDev(i) = single(fromBit_intel(344,7,Cam_obj(3:66,i)))*single(0.05)+single(0.0);
	IFC_obj_WidthStdDev(i) = single(fromBit_intel(385,7,Cam_obj(3:66,i)))*single(0.01)+single(0.0);
	IFC_obj_HeightStdDev(i) = single(fromBit_intel(297,7,Cam_obj(3:66,i)))*single(0.01)+single(0.0);
	IFC_obj_PhiLeft(i) = single(fromBit_intel(256,14,Cam_obj(3:66,i)))*single(0.0002)+single(-1.571);
	IFC_obj_PhiRight(i) = single(fromBit_intel(270,14,Cam_obj(3:66,i)))*single(0.0002)+single(-1.571);
	IFC_obj_angle_3D(i) = single(fromBit_intel(237,14,Cam_obj(3:66,i)))*single(0.0002)+single(-1.571);
	IFC_obj_PhiLeftStdDev(i) = single(fromBit_intel(224,13,Cam_obj(3:66,i)))*single(0.0002)+single(0.0);
	IFC_obj_PhiRightStdDev(i) = single(fromBit_intel(139,13,Cam_obj(3:66,i)))*single(0.0002)+single(0.0);
	IFC_obj_angle_3DStdDev(i) = single(fromBit_intel(203,13,Cam_obj(3:66,i)))*single(0.0002)+single(0.0);
	IFC_obj_angle_rate(i) = single(fromBit_intel(180,12,Cam_obj(3:66,i)))*single(0.002)+single(-2.234);
	IFC_obj_angle_rate_StdDev(i) = single(fromBit_intel(370,11,Cam_obj(3:66,i)))*single(0.002)+single(0.0);
	IFC_obj_PhiBottom(i) = single(fromBit_intel(330,14,Cam_obj(3:66,i)))*single(0.0002)+single(-1.571);
	IFC_obj_PhiBottomStdDev(i) = single(fromBit_intel(304,13,Cam_obj(3:66,i)))*single(0.0002)+single(0.0);
	IFC_obj_Measured(i) = uint8(fromBit_intel(317,2,Cam_obj(3:66,i)));
	IFC_obj_Heading(i) = single(fromBit_intel(320,10,Cam_obj(3:66,i)))*single(0.01)+single(-3.14);
	IFC_obj_HeadingStdDev(i) = single(fromBit_intel(361,9,Cam_obj(3:66,i)))*single(0.01)+single(0.0);
	IFC_obj_HeadOrientation(i) = uint8(fromBit_intel(284,4,Cam_obj(3:66,i)));
	IFC_obj_Type(i) = uint8(fromBit_intel(381,3,Cam_obj(3:66,i)));
	IFC_obj_ID(i) = uint8(fromBit_intel(392,8,Cam_obj(3:66,i)));
	IFC_obj_TTIPC(i) = single(fromBit_intel(408,11,Cam_obj(3:66,i)))*single(0.01)+single(-8.0);
	IFC_obj_TTIPC_StdDev(i) = single(fromBit_intel(401,7,Cam_obj(3:66,i)))*single(0.0625)+single(0.0);
	IFC_obj_DirIndicator(i) = uint8(fromBit_intel(253,3,Cam_obj(3:66,i)));
	IFC_obj_BrakeLight(i) = uint8(fromBit_intel(384,1,Cam_obj(3:66,i)));
	IFC_obj_timestamp(i) =  bitor(bitshift(uint16(Cam_obj(1,i)),8),uint16(Cam_obj(2,i)));
end
end

% function [IFC_State,IFC_ObjHdr_ObjCount,IFC_VD_CIPV_ID...
% ] = unpack_cam_status(IFC_Status)
% 
% IFC_State = uint8(fromBit_intel(32,4,IFC_Status(3:11)));
% IFC_ObjHdr_ObjCount = uint8(fromBit_intel(24,7,IFC_Status(3:11)));
% IFC_VD_CIPV_ID = uint8(fromBit_intel(48,8,IFC_Status(3:11)));
% end

function [IFC_State,ISA_Value,ISA_Sign_Type,ISA_Status,ISA_Popup_text,TSR_Vision_Only_Sign_Type,ADAS_IHBC_High_Beam_Req,...
    ADAS_IHBC_Fuction_Status] = unpack_cam_status(IFC_Status)
IFC_State = uint8(fromBit_motorola_onelane(24,4,IFC_Status(3:10)));
ISA_Value = uint8(fromBit_motorola_onelane(32,5,IFC_Status(3:10)));
ISA_Sign_Type = uint8(fromBit_motorola_onelane(40,3,IFC_Status(3:10)));
ISA_Status = uint8(fromBit_motorola_onelane(43,3,IFC_Status(3:10)));
ISA_Popup_text = uint8(fromBit_motorola_onelane(28,3,IFC_Status(3:10)));
TSR_Vision_Only_Sign_Type = uint8(fromBit_motorola_onelane(48,8,IFC_Status(3:10)));
ADAS_IHBC_High_Beam_Req = uint8(fromBit_motorola_onelane(6,1,IFC_Status(3:10)));
ADAS_IHBC_Fuction_Status = uint8(fromBit_motorola_onelane(4,2,IFC_Status(3:10)));
end


function [FS_Out_Of_Calib,FS_Rain,FS_Fog,FS_Splashes_0,FS_Sun_Ray_0,FS_Low_Sun_0,FS_Blur_Image_0,FS_Partial_Blockage_0,FS_Full_Blockage_0,FS_Frozen_Windshield_0,FS_Out_Of_Focus_0...
] = unpack_cam_failsafe(IFC_Failsafe)

FS_Out_Of_Calib = uint8(fromBit_intel(30,3,IFC_Failsafe(3:8)));
FS_Rain = uint8(fromBit_intel(24,3,IFC_Failsafe(3:8)));
FS_Fog = uint8(fromBit_intel(21,3,IFC_Failsafe(3:8)));
FS_Splashes_0 = uint8(fromBit_intel(15,3,IFC_Failsafe(3:8)));
FS_Sun_Ray_0 = uint8(fromBit_intel(18,3,IFC_Failsafe(3:8)));
FS_Low_Sun_0 = uint8(fromBit_intel(12,3,IFC_Failsafe(3:8)));
FS_Blur_Image_0 = uint8(fromBit_intel(9,3,IFC_Failsafe(3:8)));
FS_Partial_Blockage_0 = uint8(fromBit_intel(27,3,IFC_Failsafe(3:8)));
FS_Full_Blockage_0 = uint8(fromBit_intel(6,3,IFC_Failsafe(3:8)));
FS_Frozen_Windshield_0 = uint8(fromBit_intel(3,3,IFC_Failsafe(3:8)));
FS_Out_Of_Focus_0 = uint8(fromBit_intel(0,3,IFC_Failsafe(3:8)));
end

function [IFC_Line01_LineID,IFC_Line01_ExistProb,IFC_Line01_DxStart,IFC_Line01_ColorClass,...
    IFC_Line01_DxEnd,IFC_Line01_HeadingAngle,IFC_Line01_Dy,IFC_Line01_CurvChange,...
    IFC_Line01_Curv,IFC_Line01_MeasureType,IFC_Line01_LineWidth,IFC_Line01_Type,...
    IFC_Line01_TypeConf,IFC_Line02_LineID,IFC_Line02_ExistProb,IFC_Line02_DxStart,...
    IFC_Line02_ColorClass,IFC_Line02_DxEnd,IFC_Line02_HeadingAngle,IFC_Line02_Dy,...
    IFC_Line02_CurvChange,IFC_Line02_Curv,IFC_Line02_MeasureType,IFC_Line02_LineWidth,...
    IFC_Line02_Type,IFC_Line02_TypeConf,lane1_c1,lane2_c1...
] = unpack_cam_L0R0(IFC_L0_R0)

IFC_Line01_LineID = uint8(fromBit_intel(24,8,IFC_L0_R0(3:40)));
IFC_Line01_ExistProb = single(fromBit_intel(272,6,IFC_L0_R0(3:40)))*single(0.02)+single(0.0);
IFC_Line01_DxStart = single(fromBit_intel(128,15,IFC_L0_R0(3:40)))*single(0.01)+single(0.0);
IFC_Line01_ColorClass = uint8(fromBit_intel(84,3,IFC_L0_R0(3:40)));
IFC_Line01_DxEnd = single(fromBit_intel(32,15,IFC_L0_R0(3:40)))*single(0.01)+single(0.0);
IFC_Line01_HeadingAngle = single(fromBit_intel(111,9,IFC_L0_R0(3:40)))*single(0.01)+single(-2.0);
IFC_Line01_Dy = single(fromBit_intel(47,13,IFC_L0_R0(3:40)))*single(0.01)+single(-30.0);
IFC_Line01_CurvChange = single(fromBit_intel(64,20,IFC_L0_R0(3:40)))*single(5e-08)+single(-0.024);
IFC_Line01_Curv = single(fromBit_intel(96,15,IFC_L0_R0(3:40)))*single(1.6e-05)+single(-0.25);
IFC_Line01_MeasureType = uint8(fromBit_intel(180,2,IFC_L0_R0(3:40)));
IFC_Line01_LineWidth = single(fromBit_intel(120,7,IFC_L0_R0(3:40)))*single(0.01)+single(0.0);
IFC_Line01_Type = uint8(fromBit_intel(60,4,IFC_L0_R0(3:40)));
IFC_Line01_TypeConf = single(fromBit_intel(223,7,IFC_L0_R0(3:40)))*single(0.01)+single(0.0);
IFC_Line02_LineID = uint8(fromBit_intel(184,8,IFC_L0_R0(3:40)));
IFC_Line02_ExistProb = single(fromBit_intel(259,6,IFC_L0_R0(3:40)))*single(0.02)+single(0.0);
IFC_Line02_DxStart = single(fromBit_intel(192,15,IFC_L0_R0(3:40)))*single(0.01)+single(0.0);
IFC_Line02_ColorClass = uint8(fromBit_intel(220,3,IFC_L0_R0(3:40)));
IFC_Line02_DxEnd = single(fromBit_intel(143,15,IFC_L0_R0(3:40)))*single(0.01)+single(0.0);
IFC_Line02_HeadingAngle = single(fromBit_intel(230,9,IFC_L0_R0(3:40)))*single(0.01)+single(-2.0);
IFC_Line02_Dy = single(fromBit_intel(207,13,IFC_L0_R0(3:40)))*single(0.01)+single(-30.0);
IFC_Line02_CurvChange = single(fromBit_intel(160,20,IFC_L0_R0(3:40)))*single(5e-08)+single(-0.024);
IFC_Line02_Curv = single(fromBit_intel(240,15,IFC_L0_R0(3:40)))*single(1.6e-05)+single(-0.25);
IFC_Line02_MeasureType = uint8(fromBit_intel(278,2,IFC_L0_R0(3:40)));
IFC_Line02_LineWidth = single(fromBit_intel(265,7,IFC_L0_R0(3:40)))*single(0.01)+single(0.0);
IFC_Line02_Type = uint8(fromBit_intel(255,4,IFC_L0_R0(3:40)));
IFC_Line02_TypeConf = single(fromBit_intel(280,7,IFC_L0_R0(3:40)))*single(0.01)+single(0.0);
lane1_c1 = fromBit_intel_IEE_float(288,32,IFC_L0_R0(3:46));
lane2_c1 = fromBit_intel_IEE_float(320,32,IFC_L0_R0(3:46));
end

function [IFC_Line03_LineID,IFC_Line03_ExistProb,IFC_Line03_DxStart,IFC_Line03_ColorClass,...
    IFC_Line03_DxEnd,IFC_Line03_HeadingAngle,IFC_Line03_Dy,IFC_Line03_CurvChange,IFC_Line03_Curv,...
    IFC_Line03_MeasureType,IFC_Line03_LineWidth,IFC_Line03_Type,IFC_Line03_TypeConf,...
    IFC_Line04_LineID,IFC_Line04_ExistProb,IFC_Line04_DxStart,IFC_Line04_ColorClass,...
    IFC_Line04_DxEnd,IFC_Line04_HeadingAngle,IFC_Line04_Dy,IFC_Line04_CurvChange,IFC_Line04_Curv,...
    IFC_Line04_MeasureType,IFC_Line04_LineWidth,IFC_Line04_Type,IFC_Line04_TypeConf,...
    lane3_c1,lane4_c1...
] = unpack_cam_L1R1(IFC_L1_R1)

IFC_Line03_LineID = uint8(fromBit_intel(24,8,IFC_L1_R1(3:40)));
IFC_Line03_ExistProb = single(fromBit_intel(272,6,IFC_L1_R1(3:40)))*single(0.02)+single(0.0);
IFC_Line03_DxStart = single(fromBit_intel(128,15,IFC_L1_R1(3:40)))*single(0.01)+single(0.0);
IFC_Line03_ColorClass = uint8(fromBit_intel(84,3,IFC_L1_R1(3:40)));
IFC_Line03_DxEnd = single(fromBit_intel(32,15,IFC_L1_R1(3:40)))*single(0.01)+single(0.0);
IFC_Line03_HeadingAngle = single(fromBit_intel(111,9,IFC_L1_R1(3:40)))*single(0.01)+single(-2.0);
IFC_Line03_Dy = single(fromBit_intel(47,13,IFC_L1_R1(3:40)))*single(0.01)+single(-30.0);
IFC_Line03_CurvChange = single(fromBit_intel(64,20,IFC_L1_R1(3:40)))*single(5e-08)+single(-0.024);
IFC_Line03_Curv = single(fromBit_intel(96,15,IFC_L1_R1(3:40)))*single(1.6e-05)+single(-0.25);
IFC_Line03_MeasureType = uint8(fromBit_intel(180,2,IFC_L1_R1(3:40)));
IFC_Line03_LineWidth = single(fromBit_intel(120,7,IFC_L1_R1(3:40)))*single(0.01)+single(0.0);
IFC_Line03_Type = uint8(fromBit_intel(60,4,IFC_L1_R1(3:40)));
IFC_Line03_TypeConf = single(fromBit_intel(223,7,IFC_L1_R1(3:40)))*single(0.01)+single(0.0);
IFC_Line04_LineID = uint8(fromBit_intel(184,8,IFC_L1_R1(3:40)));
IFC_Line04_ExistProb = single(fromBit_intel(259,6,IFC_L1_R1(3:40)))*single(0.02)+single(0.0);
IFC_Line04_DxStart = single(fromBit_intel(192,15,IFC_L1_R1(3:40)))*single(0.01)+single(0.0);
IFC_Line04_ColorClass = uint8(fromBit_intel(220,3,IFC_L1_R1(3:40)));
IFC_Line04_DxEnd = single(fromBit_intel(143,15,IFC_L1_R1(3:40)))*single(0.01)+single(0.0);
IFC_Line04_HeadingAngle = single(fromBit_intel(230,9,IFC_L1_R1(3:40)))*single(0.01)+single(-2.0);
IFC_Line04_Dy = single(fromBit_intel(207,13,IFC_L1_R1(3:40)))*single(0.01)+single(-30.0);
IFC_Line04_CurvChange = single(fromBit_intel(160,20,IFC_L1_R1(3:40)))*single(5e-08)+single(-0.024);
IFC_Line04_Curv = single(fromBit_intel(240,15,IFC_L1_R1(3:40)))*single(1.6e-05)+single(-0.25);
IFC_Line04_MeasureType = uint8(fromBit_intel(278,2,IFC_L1_R1(3:40)));
IFC_Line04_LineWidth = single(fromBit_intel(265,7,IFC_L1_R1(3:40)))*single(0.01)+single(0.0);
IFC_Line04_Type = uint8(fromBit_intel(255,4,IFC_L1_R1(3:40)));
IFC_Line04_TypeConf = single(fromBit_intel(280,7,IFC_L1_R1(3:40)))*single(0.01)+single(0.0);
lane3_c1 = fromBit_intel_IEE_float(288,32,IFC_L1_R1(3:46));
lane4_c1 = fromBit_intel_IEE_float(320,32,IFC_L1_R1(3:46));
end

function [IFC_Roadedge01_LineID,IFC_Roadedge01_ExistProb,IFC_Roadedge01_DxStart,IFC_Roadedge01_DxEnd,IFC_Roadedge01_HeadingAngle,IFC_Roadedge01_Dy,IFC_Roadedge01_Curv,IFC_Roadedge01_CurvChange,IFC_Roadedge01_MeasureType,IFC_Roadedge01_Type,IFC_Roadedge02_LineID,IFC_Roadedge02_ExistProb,IFC_Roadedge02_DxStart,IFC_Roadedge02_DxEnd,IFC_Roadedge02_HeadingAngle,IFC_Roadedge02_Dy,IFC_Roadedge02_Curv,IFC_Roadedge02_CurvChange,IFC_Roadedge02_MeasureType,IFC_Roadedge02_Type...
] = unpack_cam_roadedge(IFC_Roadedge)

IFC_Roadedge01_LineID = uint8(fromBit_intel(0,8,IFC_Roadedge(3:32)));
IFC_Roadedge01_ExistProb = single(fromBit_intel(8,6,IFC_Roadedge(3:32)))*single(0.02)+single(0.0);
IFC_Roadedge01_DxStart = single(fromBit_intel(14,15,IFC_Roadedge(3:32)))*single(0.01)+single(0.0);
IFC_Roadedge01_DxEnd = single(fromBit_intel(64,15,IFC_Roadedge(3:32)))*single(0.01)+single(0.0);
IFC_Roadedge01_HeadingAngle = single(fromBit_intel(181,9,IFC_Roadedge(3:32)))*single(0.01)+single(-2.0);
IFC_Roadedge01_Dy = single(fromBit_intel(219,13,IFC_Roadedge(3:32)))*single(0.01)+single(-30.0);
IFC_Roadedge01_Curv = single(fromBit_intel(79,15,IFC_Roadedge(3:32)))*single(1.6e-05)+single(-0.25);
IFC_Roadedge01_CurvChange = single(fromBit_intel(32,20,IFC_Roadedge(3:32)))*single(5e-08)+single(-0.024);
IFC_Roadedge01_MeasureType = uint8(fromBit_intel(29,2,IFC_Roadedge(3:32)));
IFC_Roadedge01_Type = uint8(fromBit_intel(192,4,IFC_Roadedge(3:32)));
IFC_Roadedge02_LineID = uint8(fromBit_intel(56,8,IFC_Roadedge(3:32)));
IFC_Roadedge02_ExistProb = single(fromBit_intel(162,6,IFC_Roadedge(3:32)))*single(0.02)+single(0.0);
IFC_Roadedge02_DxStart = single(fromBit_intel(97,15,IFC_Roadedge(3:32)))*single(0.01)+single(0.0);
IFC_Roadedge02_DxEnd = single(fromBit_intel(112,15,IFC_Roadedge(3:32)))*single(0.01)+single(0.0);
IFC_Roadedge02_HeadingAngle = single(fromBit_intel(143,9,IFC_Roadedge(3:32)))*single(0.01)+single(-2.0);
IFC_Roadedge02_Dy = single(fromBit_intel(168,13,IFC_Roadedge(3:32)))*single(0.01)+single(-30.0);
IFC_Roadedge02_Curv = single(fromBit_intel(128,15,IFC_Roadedge(3:32)))*single(1.6e-05)+single(-0.25);
IFC_Roadedge02_CurvChange = single(fromBit_intel(196,20,IFC_Roadedge(3:32)))*single(5e-08)+single(-0.024);
IFC_Roadedge02_MeasureType = uint8(fromBit_intel(94,2,IFC_Roadedge(3:32)));
IFC_Roadedge02_Type = uint8(fromBit_intel(52,4,IFC_Roadedge(3:32)));
end
function [LH_Snown_Road_Prob,COM_Is_ghSpeed_Road_V,COM_Is_ghSpeed_Road,LAP_Is_ghway_Merge_Right,LAP_Is_ghway_Merge_Left,...
    LAP_Is_ghway_Exit_Right,LAP_Is_ghway_Exit_Left,LAP_Is_nstruction_Area] = unpack_cam_road_property(IFC_road_property)
LH_Snown_Road_Prob = single(fromBit_intel(24,7,IFC_road_property(3:9)))*single(0.01)+single(0.0);
COM_Is_ghSpeed_Road_V = uint8(fromBit_intel(38,1,IFC_road_property(3:9)));
COM_Is_ghSpeed_Road = uint8(fromBit_intel(37,1,IFC_road_property(3:9)));
LAP_Is_ghway_Merge_Right = uint8(fromBit_intel(36,1,IFC_road_property(3:9)));
LAP_Is_ghway_Merge_Left = uint8(fromBit_intel(35,1,IFC_road_property(3:9)));
LAP_Is_ghway_Exit_Right = uint8(fromBit_intel(34,1,IFC_road_property(3:9)));
LAP_Is_ghway_Exit_Left = uint8(fromBit_intel(33,1,IFC_road_property(3:9)));
LAP_Is_nstruction_Area = uint8(fromBit_intel(32,1,IFC_road_property(3:9)));
end

function [OBJ_VRUount,OBJ_VD_unt,OBJ_VD_PV_ID,OBJ_Anil_Count,AEB_VD_Alert,AEB_VD_ID,...
    AEB_VRU_Alert,AEB_VRU_PED_ID,AEBJA_VD_Alert,AEBJA_VD_ID,AEBJA_VRU_Alert,AEBJA_VRU_PED_ID,...
    AEBPrefill_VRU_Alert,AEBPrefill_VRU_PED_ID,FCW_VD_Alert,FCW_VD_ID,FCW_VRU_Alert,FCW_VRU_PED_ID,...
    JAPreFill_VD_Alert,JAPreFill_VD_ID,JAPreFill_VRU_Alert,JAPreFill_VRU_PED_ID] = unpack_cam_num_cipv(IFC_num_cipv)
OBJ_VRUount = uint8(fromBit_intel(27,5,IFC_num_cipv(3:10)));
OBJ_VD_unt = uint8(fromBit_intel(9,5,IFC_num_cipv(3:10)));
OBJ_VD_PV_ID = uint8(fromBit_intel(0,8,IFC_num_cipv(3:10)));
OBJ_Anil_Count = uint8(fromBit_intel(20,4,IFC_num_cipv(3:10)));
AEB_VD_Alert   = uint8(fromBit_intel(51,1,IFC_num_cipv(3:21)));
AEB_VD_ID  = uint8(fromBit_intel(80,8,IFC_num_cipv(3:21)));
AEB_VRU_Alert  = uint8(fromBit_intel(63,1,IFC_num_cipv(3:21)));
AEB_VRU_PED_ID  = uint8(fromBit_intel(96,8,IFC_num_cipv(3:21)));
AEBJA_VD_Alert  = uint8(fromBit_intel(48,1,IFC_num_cipv(3:21)));
AEBJA_VD_ID  = uint8(fromBit_intel(88,8,IFC_num_cipv(3:21)));
AEBJA_VRU_Alert  = uint8(fromBit_intel(56,1,IFC_num_cipv(3:21)));
AEBJA_VRU_PED_ID  = uint8(fromBit_intel(128,8,IFC_num_cipv(3:21)));
AEBPrefill_VRU_Alert  = uint8(fromBit_intel(61,1,IFC_num_cipv(3:21)));
AEBPrefill_VRU_PED_ID  = uint8(fromBit_intel(104,8,IFC_num_cipv(3:21)));
FCW_VD_Alert  = uint8(fromBit_intel(55,1,IFC_num_cipv(3:21)));
FCW_VD_ID  = uint8(fromBit_intel(64,8,IFC_num_cipv(3:21)));
FCW_VRU_Alert  = uint8(fromBit_intel(60,1,IFC_num_cipv(3:21)));
FCW_VRU_PED_ID  = uint8(fromBit_intel(112,8,IFC_num_cipv(3:21)));
JAPreFill_VD_Alert  = uint8(fromBit_intel(54,1,IFC_num_cipv(3:21)));
JAPreFill_VD_ID  = uint8(fromBit_intel(72,8,IFC_num_cipv(3:21)));
JAPreFill_VRU_Alert  = uint8(fromBit_intel(57,1,IFC_num_cipv(3:21)));
JAPreFill_VRU_PED_ID  = uint8(fromBit_intel(120,8,IFC_num_cipv(3:21)));
end
